simulink model "Navegacion"  (R2025b)
settings: Solver=VariableStepAuto  StartTime=0.0  StopTime=10.0  RelTol=1e-3
settings Model: Creator=Usuario  LastModifiedBy=Usuario

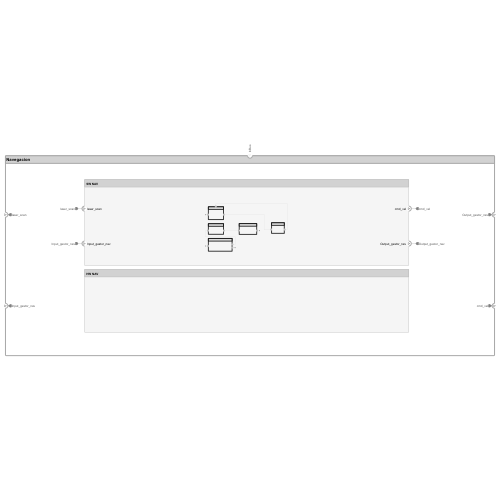
[thumbnail: Simulink's stored preview of the top-level diagram]
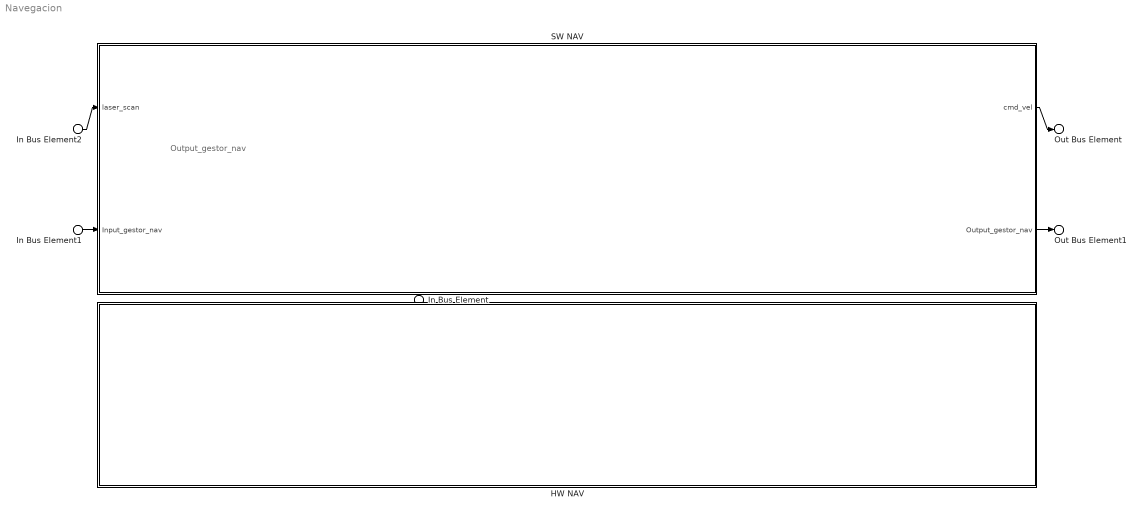
== system Navegacion ==
  note: Output_gestor_nav
  In Bus Element1 : Inport  PortName=Input_gestor_nav
  In Bus Element2 : Inport  Port=2  PortName=laser_scan
  In Bus Element : Inport  Port=3  PortName=InBus
  HW NAV : Subsystem
      settings: PortSchema="{\"entries\":[{\"content\":{\"headerSize\":26,\"margin\":15,\"minimumSpacing\":25,\"sides\":[{\"content\":{},\"type\":\"ConnectorPlacement.EquallySpacedRectSide\",\"uuid\":\"fd724ff2-3e45-4baf-8b9c-a165e1a0557a\"},{\"content\":{\"side\":\"RIGHT\"},\"type\":\"ConnectorPlacement.EquallySpacedRectSide\",\"uuid\":\"77ec35b0-ef92-4391-8d14-bb45093adaab\"},{\"content\":{\"side\":\"TOP\"},\"type\":\"ConnectorPlacement.EquallySpacedRectSide\",\"uuid\":\"f3afaf3a-e938-4dbf-8626-239eb582190a\"}]},\"type\":\"ConnectorPlacement.EquallySpacedConnector\",\"uuid\":\"512a3a62-1904-424b-ae0b-e52360ae214e\"}],\"packageUris\":[\"http://schema.mathworks.com/mf0/Connector/R2020b\"],\"version\":\"1.0\"}"
  SW NAV : Subsystem
      settings: PortSchema="{\"entries\":[{\"content\":{\"headerSize\":26,\"margin\":15,\"minimumSpacing\":25,\"sides\":[{\"content\":{\"connectorIds\":[\"In1\",\"In2\"]},\"type\":\"ConnectorPlacement.EquallySpacedRectSide\",\"uuid\":\"fd724ff2-3e45-4baf-8b9c-a165e1a0557a\"},{\"content\":{\"connectorIds\":[\"Out1\",\"Out2\"],\"side\":\"RIGHT\"},\"type\":\"ConnectorPlacement.EquallySpacedRectSide\",\"uuid\":\"77ec35b0-ef92-4391-8d14-bb45093adaab\"},{\"content\":{\"side\":\"TOP\"},\"type\":\"ConnectorPlacement.EquallySpacedRectSide\",\"uuid\":\"f3afaf3a-e938-4dbf-8626-239eb582190a\"}]},\"type\":\"ConnectorPlacement.EquallySpacedConnector\",\"uuid\":\"512a3a62-1904-424b-ae0b-e52360ae214e\"}],\"packageUris\":[\"http://schema.mathworks.com/mf0/Connector/R2020b\"],\"version\":\"1.0\"}"
  Out Bus Element1 : Outport  PortName=Output_gestor_nav
  Out Bus Element : Outport  Port=2  PortName=cmd_vel
  wires:
  In Bus Element2/1 -> SW NAV/1(laser_scan)
  In Bus Element1/1 -> SW NAV/2(Input_gestor_nav)
  SW NAV/1(cmd_vel) -> Out Bus Element/1
  SW NAV/2(Output_gestor_nav) -> Out Bus Element1/1

== system Navegacion/HW NAV ==

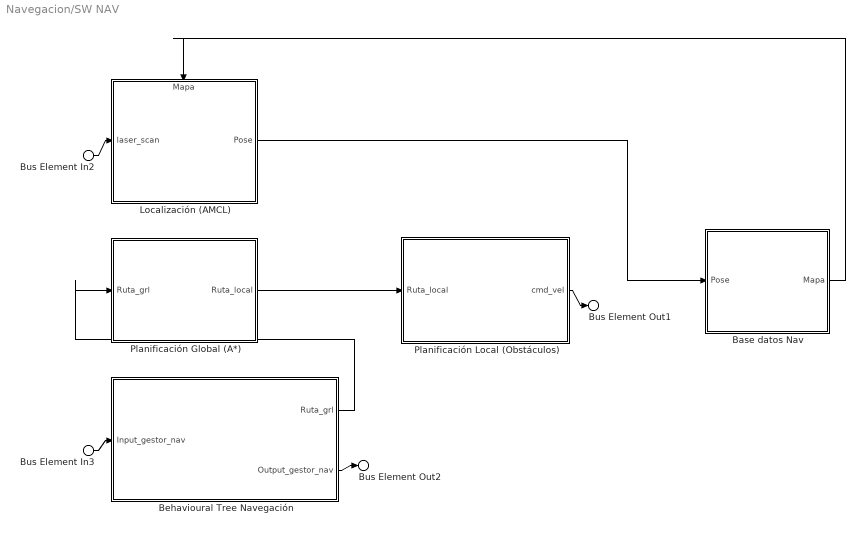
== system Navegacion/SW NAV ==
  Bus Element In2 : Inport  PortName=laser_scan
  Bus Element In3 : Inport  Port=2  PortName=Input_gestor_nav
  Base datos Nav : Subsystem
      settings: PortSchema="{\"entries\":[{\"content\":{\"headerSize\":26,\"margin\":15,\"minimumSpacing\":25,\"sides\":[{\"content\":{\"connectorIds\":[\"In1\"]},\"type\":\"ConnectorPlacement.EquallySpacedRectSide\",\"uuid\":\"fd724ff2-3e45-4baf-8b9c-a165e1a0557a\"},{\"content\":{\"connectorIds\":[\"Out1\"],\"side\":\"RIGHT\"},\"type\":\"ConnectorPlacement.EquallySpacedRectSide\",\"uuid\":\"77ec35b0-ef92-4391-8d14-bb45093adaab\"},{\"content\":{\"side\":\"TOP\"},\"type\":\"ConnectorPlacement.EquallySpacedRectSide\",\"uuid\":\"f3afaf3a-e938-4dbf-8626-239eb582190a\"}]},\"type\":\"ConnectorPlacement.EquallySpacedConnector\",\"uuid\":\"512a3a62-1904-424b-ae0b-e52360ae214e\"}],\"packageUris\":[\"http://schema.mathworks.com/mf0/Connector/R2020b\"],\"version\":\"1.0\"}"
  Behavioural Tree Navegación : Subsystem
      settings: PortSchema="{\"entries\":[{\"content\":{\"headerSize\":26,\"margin\":15,\"minimumSpacing\":25,\"sides\":[{\"content\":{\"connectorIds\":[\"In1\"]},\"type\":\"ConnectorPlacement.EquallySpacedRectSide\",\"uuid\":\"fd724ff2-3e45-4baf-8b9c-a165e1a0557a\"},{\"content\":{\"connectorIds\":[\"Out1\",\"Out2\"],\"side\":\"RIGHT\"},\"type\":\"ConnectorPlacement.EquallySpacedRectSide\",\"uuid\":\"77ec35b0-ef92-4391-8d14-bb45093adaab\"},{\"content\":{\"side\":\"TOP\"},\"type\":\"ConnectorPlacement.EquallySpacedRectSide\",\"uuid\":\"f3afaf3a-e938-4dbf-8626-239eb582190a\"}]},\"type\":\"ConnectorPlacement.EquallySpacedConnector\",\"uuid\":\"512a3a62-1904-424b-ae0b-e52360ae214e\"}],\"packageUris\":[\"http://schema.mathworks.com/mf0/Connector/R2020b\"],\"version\":\"1.0\"}"
  Localización (AMCL) : Subsystem
      settings: PortSchema="{\"entries\":[{\"content\":{\"headerSize\":26,\"margin\":15,\"minimumSpacing\":25,\"sides\":[{\"content\":{\"connectorIds\":[\"In1\"]},\"type\":\"ConnectorPlacement.EquallySpacedRectSide\",\"uuid\":\"fd724ff2-3e45-4baf-8b9c-a165e1a0557a\"},{\"content\":{\"connectorIds\":[\"Out1\"],\"side\":\"RIGHT\"},\"type\":\"ConnectorPlacement.EquallySpacedRectSide\",\"uuid\":\"77ec35b0-ef92-4391-8d14-bb45093adaab\"},{\"content\":{\"connectorIds\":[\"In2\"],\"side\":\"TOP\"},\"type\":\"ConnectorPlacement.EquallySpacedRectSide\",\"uuid\":\"f3afaf3a-e938-4dbf-8626-239eb582190a\"}]},\"type\":\"ConnectorPlacement.EquallySpacedConnector\",\"uuid\":\"512a3a62-1904-424b-ae0b-e52360ae214e\"}],\"packageUris\":[\"http://schema.mathworks.com/mf0/Connector/R2020b\"],\"version\":\"1.0\"}"
  Planificación Global (A*) : Subsystem
      settings: PortSchema="{\"entries\":[{\"content\":{\"headerSize\":26,\"margin\":15,\"minimumSpacing\":25,\"sides\":[{\"content\":{\"connectorIds\":[\"In1\"]},\"type\":\"ConnectorPlacement.EquallySpacedRectSide\",\"uuid\":\"fd724ff2-3e45-4baf-8b9c-a165e1a0557a\"},{\"content\":{\"connectorIds\":[\"Out1\"],\"side\":\"RIGHT\"},\"type\":\"ConnectorPlacement.EquallySpacedRectSide\",\"uuid\":\"77ec35b0-ef92-4391-8d14-bb45093adaab\"},{\"content\":{\"side\":\"TOP\"},\"type\":\"ConnectorPlacement.EquallySpacedRectSide\",\"uuid\":\"f3afaf3a-e938-4dbf-8626-239eb582190a\"}]},\"type\":\"ConnectorPlacement.EquallySpacedConnector\",\"uuid\":\"512a3a62-1904-424b-ae0b-e52360ae214e\"}],\"packageUris\":[\"http://schema.mathworks.com/mf0/Connector/R2020b\"],\"version\":\"1.0\"}"
  Planificación Local (Obstáculos) : Subsystem
      settings: PortSchema="{\"entries\":[{\"content\":{\"headerSize\":26,\"margin\":15,\"minimumSpacing\":25,\"sides\":[{\"content\":{\"connectorIds\":[\"In1\"]},\"type\":\"ConnectorPlacement.EquallySpacedRectSide\",\"uuid\":\"fd724ff2-3e45-4baf-8b9c-a165e1a0557a\"},{\"content\":{\"connectorIds\":[\"Out1\"],\"side\":\"RIGHT\"},\"type\":\"ConnectorPlacement.EquallySpacedRectSide\",\"uuid\":\"77ec35b0-ef92-4391-8d14-bb45093adaab\"},{\"content\":{\"side\":\"TOP\"},\"type\":\"ConnectorPlacement.EquallySpacedRectSide\",\"uuid\":\"f3afaf3a-e938-4dbf-8626-239eb582190a\"}]},\"type\":\"ConnectorPlacement.EquallySpacedConnector\",\"uuid\":\"512a3a62-1904-424b-ae0b-e52360ae214e\"}],\"packageUris\":[\"http://schema.mathworks.com/mf0/Connector/R2020b\"],\"version\":\"1.0\"}"
  Bus Element Out1 : Outport  PortName=cmd_vel
  Bus Element Out2 : Outport  Port=2  PortName=Output_gestor_nav
  wires:
  Localización (AMCL)/1(Pose) -> Base datos Nav/1(Pose)
  Base datos Nav/1(Mapa) -> Localización (AMCL)/2(Mapa)
  Behavioural Tree Navegación/1(Ruta_grl) -> Planificación Global (A*)/1(Ruta_grl)
  Planificación Global (A*)/1(Ruta_local) -> Planificación Local (Obstáculos)/1(Ruta_local)
  Planificación Local (Obstáculos)/1(cmd_vel) -> Bus Element Out1/1
  Bus Element In2/1 -> Localización (AMCL)/1(laser_scan)
  Bus Element In3/1 -> Behavioural Tree Navegación/1(Input_gestor_nav)
  Behavioural Tree Navegación/2(Output_gestor_nav) -> Bus Element Out2/1

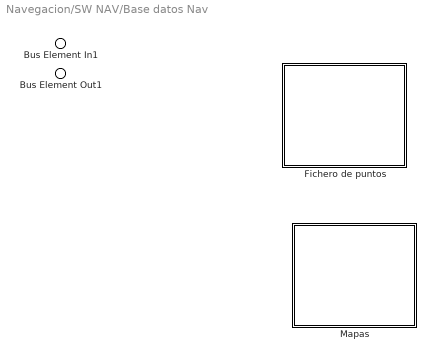
== system Navegacion/SW NAV/Base datos Nav ==
  Bus Element In1 : Inport  PortName=Pose
  Fichero de puntos : Subsystem
      settings: PortSchema="{\"entries\":[{\"content\":{\"headerSize\":26,\"margin\":15,\"minimumSpacing\":25,\"sides\":[{\"content\":{},\"type\":\"ConnectorPlacement.EquallySpacedRectSide\",\"uuid\":\"fd724ff2-3e45-4baf-8b9c-a165e1a0557a\"},{\"content\":{\"side\":\"RIGHT\"},\"type\":\"ConnectorPlacement.EquallySpacedRectSide\",\"uuid\":\"77ec35b0-ef92-4391-8d14-bb45093adaab\"},{\"content\":{\"side\":\"TOP\"},\"type\":\"ConnectorPlacement.EquallySpacedRectSide\",\"uuid\":\"f3afaf3a-e938-4dbf-8626-239eb582190a\"}]},\"type\":\"ConnectorPlacement.EquallySpacedConnector\",\"uuid\":\"512a3a62-1904-424b-ae0b-e52360ae214e\"}],\"packageUris\":[\"http://schema.mathworks.com/mf0/Connector/R2020b\"],\"version\":\"1.0\"}"
  Mapas : Subsystem
      settings: PortSchema="{\"entries\":[{\"content\":{\"headerSize\":26,\"margin\":15,\"minimumSpacing\":25,\"sides\":[{\"content\":{},\"type\":\"ConnectorPlacement.EquallySpacedRectSide\",\"uuid\":\"fd724ff2-3e45-4baf-8b9c-a165e1a0557a\"},{\"content\":{\"side\":\"RIGHT\"},\"type\":\"ConnectorPlacement.EquallySpacedRectSide\",\"uuid\":\"77ec35b0-ef92-4391-8d14-bb45093adaab\"},{\"content\":{\"side\":\"TOP\"},\"type\":\"ConnectorPlacement.EquallySpacedRectSide\",\"uuid\":\"f3afaf3a-e938-4dbf-8626-239eb582190a\"}]},\"type\":\"ConnectorPlacement.EquallySpacedConnector\",\"uuid\":\"512a3a62-1904-424b-ae0b-e52360ae214e\"}],\"packageUris\":[\"http://schema.mathworks.com/mf0/Connector/R2020b\"],\"version\":\"1.0\"}"
  Bus Element Out1 : Outport  PortName=Mapa

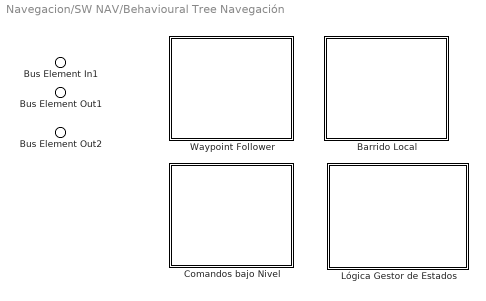
== system Navegacion/SW NAV/Behavioural Tree Navegación ==
  Bus Element In1 : Inport  PortName=Input_gestor_nav
  Barrido Local : Subsystem
      settings: PortSchema="{\"entries\":[{\"content\":{\"headerSize\":26,\"margin\":15,\"minimumSpacing\":25,\"sides\":[{\"content\":{},\"type\":\"ConnectorPlacement.EquallySpacedRectSide\",\"uuid\":\"fd724ff2-3e45-4baf-8b9c-a165e1a0557a\"},{\"content\":{\"side\":\"RIGHT\"},\"type\":\"ConnectorPlacement.EquallySpacedRectSide\",\"uuid\":\"77ec35b0-ef92-4391-8d14-bb45093adaab\"},{\"content\":{\"side\":\"TOP\"},\"type\":\"ConnectorPlacement.EquallySpacedRectSide\",\"uuid\":\"f3afaf3a-e938-4dbf-8626-239eb582190a\"}]},\"type\":\"ConnectorPlacement.EquallySpacedConnector\",\"uuid\":\"512a3a62-1904-424b-ae0b-e52360ae214e\"}],\"packageUris\":[\"http://schema.mathworks.com/mf0/Connector/R2020b\"],\"version\":\"1.0\"}"
  Comandos bajo Nivel : Subsystem
      settings: PortSchema="{\"entries\":[{\"content\":{\"headerSize\":26,\"margin\":15,\"minimumSpacing\":25,\"sides\":[{\"content\":{},\"type\":\"ConnectorPlacement.EquallySpacedRectSide\",\"uuid\":\"fd724ff2-3e45-4baf-8b9c-a165e1a0557a\"},{\"content\":{\"side\":\"RIGHT\"},\"type\":\"ConnectorPlacement.EquallySpacedRectSide\",\"uuid\":\"77ec35b0-ef92-4391-8d14-bb45093adaab\"},{\"content\":{\"side\":\"TOP\"},\"type\":\"ConnectorPlacement.EquallySpacedRectSide\",\"uuid\":\"f3afaf3a-e938-4dbf-8626-239eb582190a\"}]},\"type\":\"ConnectorPlacement.EquallySpacedConnector\",\"uuid\":\"512a3a62-1904-424b-ae0b-e52360ae214e\"}],\"packageUris\":[\"http://schema.mathworks.com/mf0/Connector/R2020b\"],\"version\":\"1.0\"}"
  Lógica Gestor de Estados : Subsystem
      settings: PortSchema="{\"entries\":[{\"content\":{\"headerSize\":26,\"margin\":15,\"minimumSpacing\":25,\"sides\":[{\"content\":{},\"type\":\"ConnectorPlacement.EquallySpacedRectSide\",\"uuid\":\"fd724ff2-3e45-4baf-8b9c-a165e1a0557a\"},{\"content\":{\"side\":\"RIGHT\"},\"type\":\"ConnectorPlacement.EquallySpacedRectSide\",\"uuid\":\"77ec35b0-ef92-4391-8d14-bb45093adaab\"},{\"content\":{\"side\":\"TOP\"},\"type\":\"ConnectorPlacement.EquallySpacedRectSide\",\"uuid\":\"f3afaf3a-e938-4dbf-8626-239eb582190a\"}]},\"type\":\"ConnectorPlacement.EquallySpacedConnector\",\"uuid\":\"512a3a62-1904-424b-ae0b-e52360ae214e\"}],\"packageUris\":[\"http://schema.mathworks.com/mf0/Connector/R2020b\"],\"version\":\"1.0\"}"
  Waypoint Follower : Subsystem
      settings: PortSchema="{\"entries\":[{\"content\":{\"headerSize\":26,\"margin\":15,\"minimumSpacing\":25,\"sides\":[{\"content\":{},\"type\":\"ConnectorPlacement.EquallySpacedRectSide\",\"uuid\":\"fd724ff2-3e45-4baf-8b9c-a165e1a0557a\"},{\"content\":{\"side\":\"RIGHT\"},\"type\":\"ConnectorPlacement.EquallySpacedRectSide\",\"uuid\":\"77ec35b0-ef92-4391-8d14-bb45093adaab\"},{\"content\":{\"side\":\"TOP\"},\"type\":\"ConnectorPlacement.EquallySpacedRectSide\",\"uuid\":\"f3afaf3a-e938-4dbf-8626-239eb582190a\"}]},\"type\":\"ConnectorPlacement.EquallySpacedConnector\",\"uuid\":\"512a3a62-1904-424b-ae0b-e52360ae214e\"}],\"packageUris\":[\"http://schema.mathworks.com/mf0/Connector/R2020b\"],\"version\":\"1.0\"}"
  Bus Element Out1 : Outport  PortName=Ruta_grl
  Bus Element Out2 : Outport  Port=2  PortName=Output_gestor_nav

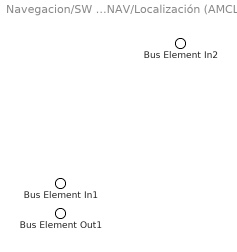
== system Navegacion/SW NAV/Localización (AMCL) ==
  Bus Element In2 : Inport  PortName=laser_scan
  Bus Element In1 : Inport  Port=2  PortName=Mapa
  Bus Element Out1 : Outport  PortName=Pose

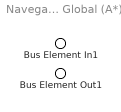
== system Navegacion/SW NAV/Planificación Global (A*) ==
  Bus Element In1 : Inport  PortName=Ruta_grl
  Bus Element Out1 : Outport  PortName=Ruta_local

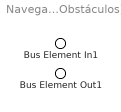
== system Navegacion/SW NAV/Planificación Local (Obstáculos) ==
  Bus Element In1 : Inport  PortName=Ruta_local
  Bus Element Out1 : Outport  PortName=cmd_vel

== system Navegacion/SW NAV/Base datos Nav/Fichero de puntos ==

== system Navegacion/SW NAV/Base datos Nav/Mapas ==

== system Navegacion/SW NAV/Behavioural Tree Navegación/Barrido Local ==

== system Navegacion/SW NAV/Behavioural Tree Navegación/Comandos bajo Nivel ==

== system Navegacion/SW NAV/Behavioural Tree Navegación/Lógica Gestor de Estados ==

== system Navegacion/SW NAV/Behavioural Tree Navegación/Waypoint Follower ==
